simulink model "KF_3D_linear_sim"  (R2016b)
settings: Solver=FixedStepAuto  StartTime=0.0  StopTime=100  FixedStep=0.001  RelTol=1e-3
values from neighbouring files (symbols this model uses):
  A = [0, 1, 0; (m*g*l_C)/I_G, (-C_phi-C_psi)/I_G, C_psi/I_G; 0, C_psi/I_R, -C_psi/I_R]    [Beobachter_1D_diskret.m]    (also in Beobachter_3D_diskret.m = [zeros(3,3), g_LA, zeros(3,3); KF_3D_linear.m = minSYS.A)
  B = [0; -1/I_G; 1/I_R]    [Beobachter_1D_diskret.m]    (also in Beobachter_3D_diskret.m = [zeros(3,3); -I_K_inv; I_R_inv]; KF_3D_linear.m = minSYS.B)
  C = [0, 1, 0;0,0,1]    [Beobachter_1D_diskret.m]    (also in Beobachter_3D_diskret.m = [zeros(3,3),eye(3), zeros(3,3); KF_3D_linear.m = minSYS.C)
  Kd = lqrd(minSYS.A, minSYS.B, Q, R, 0.02)    [Beobachter_3D_diskret.m]
  T_red = [eye(7), zeros(7,2)]    [Beobachter_3D_diskret.m]
  Ta = 0.02    [Beobachter_1D_diskret.m]    (also in KF_3D_linear.m)
  x_0 = degtorad([5;0;0])    [Beobachter_1D_diskret.m]    (also in KF_3D_linear.m = [ [-6.3118;-4.9313;-5.6638]+9.81/sqrt(3);zeros(6,1) ])
undefined symbols (not defined in the file or in its folder): Ad_K, Bd_K, Cd_K, Ld_K, T_K
settings Model: Creator=michael  LastModifiedBy=michael

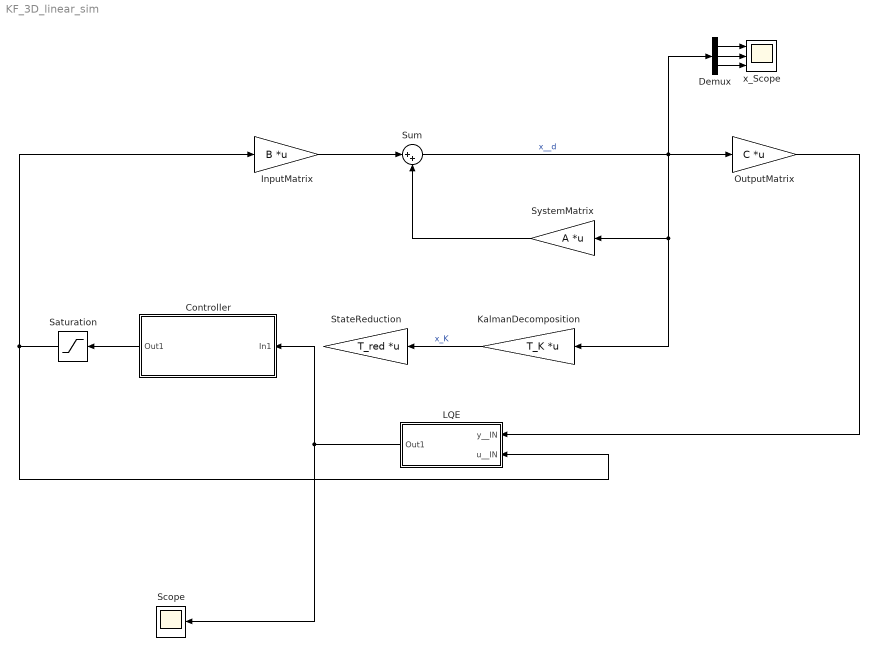
== system KF_3D_linear_sim ==
  Controller : Subsystem
  Demux : Demux  Outputs=3
  InputMatrix : Gain  Gain=B  Multiplication=Matrix(K*u) (u vector)
  KalmanDecomposition : Gain  Gain=T_K  Multiplication=Matrix(K*u) (u vector)
  LQE : Subsystem
  OutputMatrix : Gain  Gain=C  Multiplication=Matrix(K*u) (u vector)
  Saturation : Saturate  UpperLimit=0.13  LowerLimit=-0.13
  Scope : Scope
  StateReduction : Gain  Gain=T_red  Multiplication=Matrix(K*u) (u vector)
  Sum : Sum  Inputs=|++
  SystemMatrix : Gain  Gain=A  Multiplication=Matrix(K*u) (u vector)
  x_Scope : Scope  NumInputPorts=3
  wires:
  Sum/1 -> Demux/1, OutputMatrix/1, SystemMatrix/1, KalmanDecomposition/1  "x__d"
  SystemMatrix/1 -> Sum/2
  InputMatrix/1 -> Sum/1
  Demux/1 -> x_Scope/1
  Demux/2 -> x_Scope/2
  Demux/3 -> x_Scope/3
  OutputMatrix/1 -> LQE/1(y__IN)
  Controller/1(Out1) -> Saturation/1
  Saturation/1 -> LQE/2(u__IN), InputMatrix/1
  KalmanDecomposition/1 -> StateReduction/1  "x_K"
  LQE/1(Out1) -> Scope/1, Controller/1(In1)

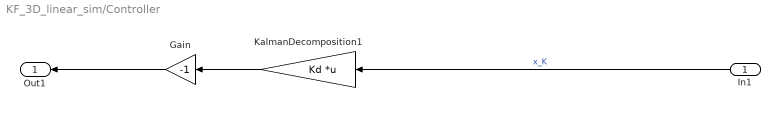
== system KF_3D_linear_sim/Controller ==
  In1 : Inport  SampleTime=Ta
  Gain : Gain  Gain=-1
  KalmanDecomposition1 : Gain  Gain=Kd  Multiplication=Matrix(K*u) (u vector)
  Out1 : Outport
  wires:
  Gain/1 -> Out1/1
  KalmanDecomposition1/1 -> Gain/1
  In1/1 -> KalmanDecomposition1/1  "x_K"

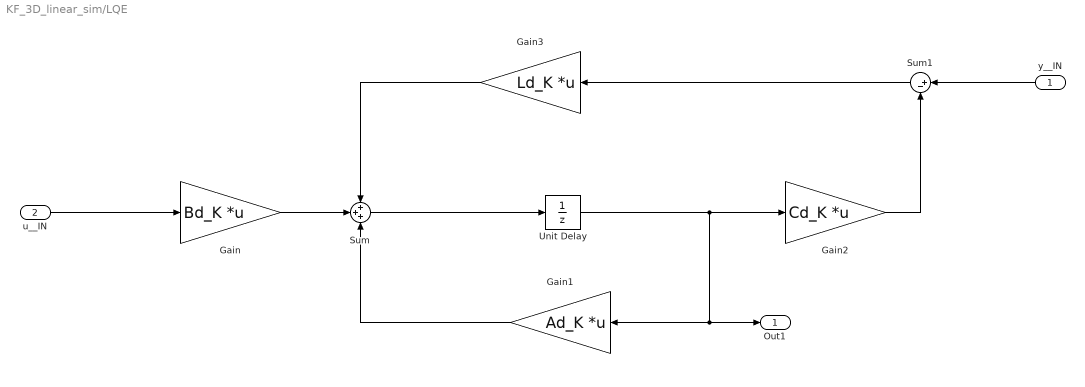
== system KF_3D_linear_sim/LQE ==
  y__IN : Inport
  u__IN : Inport  Port=2
  Gain : Gain  Gain=Bd_K  Multiplication=Matrix(K*u) (u vector)
  Gain1 : Gain  Gain=Ad_K  Multiplication=Matrix(K*u) (u vector)
  Gain2 : Gain  Gain=Cd_K  Multiplication=Matrix(K*u) (u vector)
  Gain3 : Gain  Gain=Ld_K  Multiplication=Matrix(K*u) (u vector)
  Sum : Sum  Inputs=+++
  Sum1 : Sum  Inputs=|+-
  Unit Delay : UnitDelay  InitialCondition=T_red*T_K*x_0  SampleTime=Ta
  Out1 : Outport
  wires:
  u__IN/1 -> Gain/1
  Sum/1 -> Unit Delay/1
  Gain1/1 -> Sum/3
  Unit Delay/1 -> Gain1/1, Out1/1, Gain2/1
  Gain/1 -> Sum/2
  Gain3/1 -> Sum/1
  Sum1/1 -> Gain3/1
  Gain2/1 -> Sum1/2
  y__IN/1 -> Sum1/1
